simulink model "Simulation_Problem2b"  (R2024a)
settings: Solver=VariableStepAuto  StartTime=0.0  StopTime=10.0  RelTol=1e-3
settings Model: Creator=hp  LastModifiedBy=hp

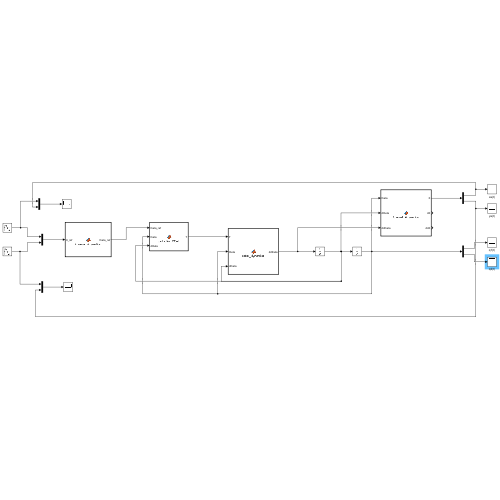
[thumbnail: Simulink's stored preview of the top-level diagram]
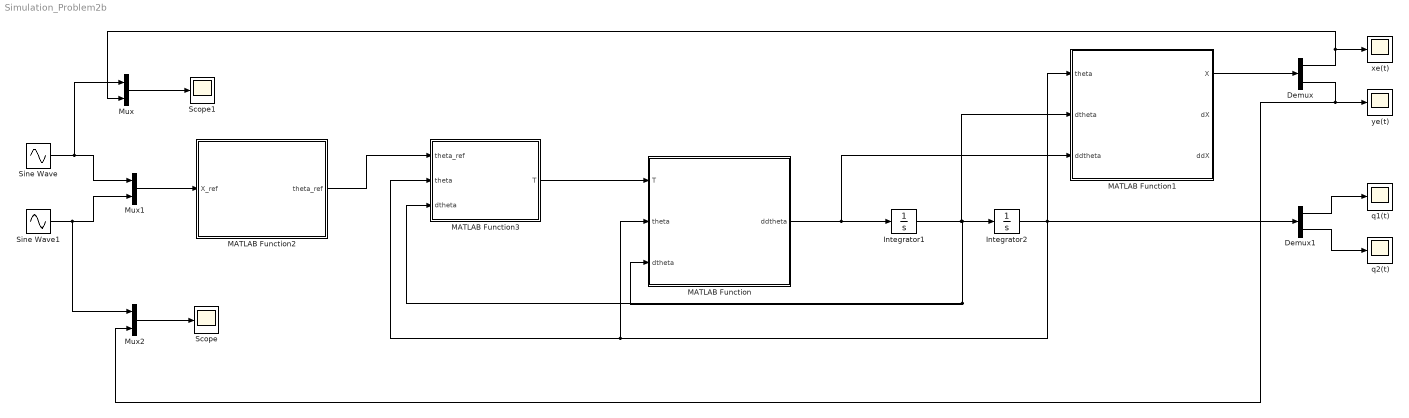
== system Simulation_Problem2b ==
  Demux : Demux  Outputs=2
  Demux1 : Demux  Outputs=2
  Integrator1 : Integrator  InitialCondition=[0; 0]
  Integrator2 : Integrator  InitialCondition=[0; 0]
  MATLAB Function : MATLAB Function  TreatAsAtomicUnit=on
  MATLAB Function1 : MATLAB Function  TreatAsAtomicUnit=on
  MATLAB Function2 : MATLAB Function  TreatAsAtomicUnit=on
  MATLAB Function3 : MATLAB Function  TreatAsAtomicUnit=on
  Mux : Mux  Inputs=2
  Mux1 : Mux  Inputs=2
  Mux2 : Mux  Inputs=2
  Scope : Scope
  Scope1 : Scope
  Sine Wave : Sin  Amplitude=0.16  Bias=0.59  Frequency=2  SampleTime=0
  Sine Wave1 : Sin  Amplitude=0.16  Bias=0.59  Frequency=3  SampleTime=0
  q1(t) : Scope
  q2(t) : Scope
  xe(t) : Scope
  ye(t) : Scope
  wires:
  Sine Wave/1 -> Mux/1, Mux1/1
  MATLAB Function1/1(X) -> Demux/1
  Mux/1 -> Scope1/1
  Sine Wave1/1 -> Mux2/1, Mux1/2
  Demux1/2 -> q2(t)/1
  Integrator2/1 -> Demux1/1, MATLAB Function1/1(theta), MATLAB Function3/2(theta), MATLAB Function/2(theta)
  Integrator1/1 -> MATLAB Function1/2(dtheta), MATLAB Function3/3(dtheta), MATLAB Function/3(dtheta), Integrator2/1
  Demux/2 -> Mux2/2, ye(t)/1
  MATLAB Function/1(ddtheta) -> MATLAB Function1/3(ddtheta), Integrator1/1
  MATLAB Function3/1(T) -> MATLAB Function/1(T)
  Demux1/1 -> q1(t)/1
  Demux/1 -> Mux/2, xe(t)/1
  Mux1/1 -> MATLAB Function2/1(X_ref)
  MATLAB Function2/1(theta_ref) -> MATLAB Function3/1(theta_ref)
  Mux2/1 -> Scope/1

== matlab function Simulation_Problem2b/MATLAB Function1 ==
  data: theta input; X output; dtheta input; ddtheta input; dX output; ddX output
function [X, dX, ddX] = forward_kinematics(theta, dtheta, ddtheta)
% Ileri Kinematik ve Jacobian Hesaplamalari
% Problem 1 - Uç Nokta Degerleri

% l1 ve l2 degerleri
l1 = 0.83; 
l2 = 0.46;

th1 = theta(1); th2 = theta(2);
dth1 = dtheta(1); dth2 = dtheta(2);
ddth1 = ddtheta(1); ddth2 = ddtheta(2);

% 1. Konum (X)
xe = l1*cos(th1) + l2*cos(th1+th2);
ye = l1*sin(th1) + l2*sin(th1+th2);
X = [xe; ye];

% 2. Jacobian Matrisi ve Hiz (dX)
J11 = -l1*sin(th1) - l2*sin(th1+th2);
J12 = -l2*sin(th1+th2);
J21 = l1*cos(th1) + l2*cos(th1+th2);
J22 = l2*cos(th1+th2);
J = [J11, J12; J21, J22];

dX = J * [dth1; dth2];

% 3. Jacobian Turevi ve Ivme (ddX)
dJ11 = -l1*cos(th1)*dth1 - l2*cos(th1+th2)*(dth1+dth2);
dJ12 = -l2*cos(th1+th2)*(dth1+dth2);
dJ21 = -l1*sin(th1)*dth1 - l2*sin(th1+th2)*(dth1+dth2);
dJ22 = -l2*sin(th1+th2)*(dth1+dth2);
dJ = [dJ11, dJ12; dJ21, dJ22];

ddX = dJ * [dth1; dth2] + J * [ddth1; ddth2];
end

== matlab function Simulation_Problem2b/MATLAB Function ==
  data: T input; ddtheta output; theta input; dtheta input
function ddtheta = robot_dynamics(T, theta, dtheta)
% Problem 1 - Dinamik Model

% Kendi grubumuzun degerlerini garanti olsun diye buraya da yaziyoruz 
% (Simulink'in Workspace'den cekerken hata vermesini engellemek icin)
l1 = 0.83; l2 = 0.46;
r1 = 0.42; r2 = 0.23;
m1 = 0.66; m2 = 0.37;
I1 = 0.03; I2 = 0.02;
g = 9.81;

th1 = theta(1); th2 = theta(2);
dth1 = dtheta(1); dth2 = dtheta(2);
T1 = T(1); T2 = T(2);

% A(theta) Matrisi Parametreleri
a11 = m2*l1^2 + 2*m2*l1*r2*cos(th2) + m1*r1^2 + m2*r2^2 + I1 + I2; 
a12 = m2*r2^2 + l1*m2*r2*cos(th2) + I2; 
a21 = m2*r2^2 + l1*m2*r2*cos(th2) + I2; 
a22 = m2*r2^2 + I2; 
A = [a11, a12; a21, a22]; 

% B(theta, dtheta) Matrisi Parametreleri
b11 = -2*l1*m2*r2*sin(th2)*dth2; 
b12 = -2*l1*m2*r2*sin(th2)*dth1 - 2*l1*m2*r2*sin(th2)*dth2; 
b21 = 2*l1*m2*r2*sin(th2)*dth1; 
b22 = 0; 
B = [b11, b12; b21, b22]; 

% G(theta) Matrisi Parametreleri
g1 = m2*r2*g*cos(th1+th2) + m2*l1*g*cos(th1) + m1*r1*g*cos(th1); 
g2 = m2*r2*g*cos(th1+th2); 
G = [g1; g2]; 

% Tork Vektoru
Tau = [T1; T2];

% Dinamik Denklemin Cozumu
ddtheta = A \ (Tau - B*dtheta - G); 
end

== matlab function Simulation_Problem2b/MATLAB Function2 ==
  data: X_ref input; theta_ref output
function theta_ref = inverse_kinematics(X_ref)

l1 = 0.83; 
l2 = 0.46;
xe = X_ref(1);
ye = X_ref(2);

% D formulu
D = (xe^2 + ye^2 - l1^2 - l2^2) / (2*l1*l2);

% Fiziksel sinirlari asmamasi icin guvenlik onlemi (D degeri -1 ile 1 arasinda olmalidir)
if D > 1
    D = 1;
elseif D < -1
    D = -1;
end

% Aci formulleri
th2_ref = atan2(sqrt(1-D^2), D);
th1_ref = atan2(ye, xe) - atan2(l2*sin(th2_ref), l1 + l2*cos(th2_ref));

theta_ref = [th1_ref; th2_ref];
end

== matlab function Simulation_Problem2b/MATLAB Function3 ==
  data: theta_ref input; T output; theta input; dtheta input
function T = controller_DOob(theta_ref, theta, dtheta)
% Problem 2 - Konum Kontrolcusu ve Gozlemci 

% Grubun Degerleri
l1 = 0.83; l2 = 0.46;
r1 = 0.42; r2 = 0.23;
m1 = 0.66; m2 = 0.37;
I1 = 0.03; I2 = 0.02;
g = 9.81;

% PD Kontrol Katsayilari
Kp = 150;
Kd = 30;

th1 = theta(1); th2 = theta(2);
dth1 = dtheta(1); dth2 = dtheta(2);

% 1. Adim: PD Konum Kontrolcusu (Sadece ivme referansi uretir)
ddtheta_ref = Kp * (theta_ref - theta) - Kd * dtheta;

% 2. Adim: Dinamik Model / Gozlemci Kompanzasyonu
a11 = m2*l1^2 + 2*m2*l1*r2*cos(th2) + m1*r1^2 + m2*r2^2 + I1 + I2;
a12 = m2*r2^2 + l1*m2*r2*cos(th2) + I2;
a21 = m2*r2^2 + l1*m2*r2*cos(th2) + I2;
a22 = m2*r2^2 + I2;
A = [a11, a12; a21, a22];

b11 = -2*l1*m2*r2*sin(th2)*dth2;
b12 = -2*l1*m2*r2*sin(th2)*dth1 - 2*l1*m2*r2*sin(th2)*dth2;
b21 = 2*l1*m2*r2*sin(th2)*dth1;
b22 = 0;
B = [b11, b12; b21, b22];

g1 = m2*r2*g*cos(th1+th2) + m2*l1*g*cos(th1) + m1*r1*g*cos(th1);
g2 = m2*r2*g*cos(th1+th2);
G = [g1; g2];

% Motorlara gidecek nihai Tork (T = A*ddtheta_ref + B*dtheta + G)
T = A * ddtheta_ref + B * dtheta + G;
end
